simulink model "ED_PROJ"  (R2016a)
settings: Solver=VariableStepAuto  StartTime=0.0  StopTime=2  RelTol=1e-3
libraries: powerlib x12, simulink x1
settings Model: Creator=Deepak  LastModifiedBy=Deepak

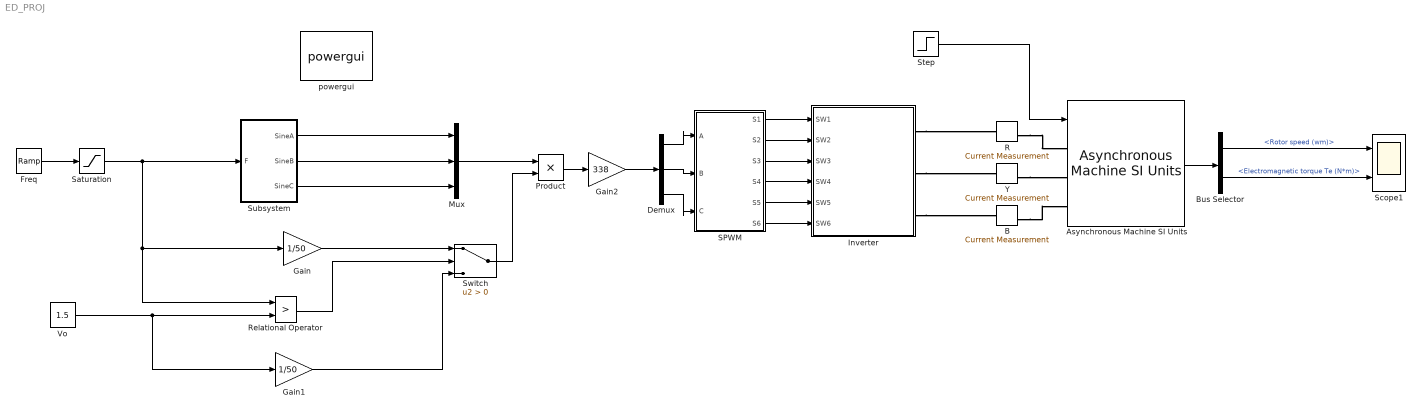
== system ED_PROJ ==
  Asynchronous Machine SI Units : powerlib/Machines/Asynchronous Machine SI Units  RotorType=Squirrel-cage  PresetModel=No  MechanicalLoad=Torque Tm  ShowDetailedParameters=on  ReferenceFrame=Rotor  Units=SI  MeasurementBus=off  NominalParameters=[1.845e+04 415 50]  Stator=[0.5968 0.0003495]  Rotor=[0.6258 0.005473]  Cage1=[0.4155 0.002066]  Cage2=[0.4168 0.0003495]  Lm=0.0354  Mechanical=[0.05 0.005879 2]  PolePairs=2  InitialConditions=[1 0 0 0 0 0 0 0]  SimulateSaturation=off  Saturation=[14.03593122, 27.81365428, 53.79336849, 72.68890987, 97.98006896, 148.6815601, 215.7428561, 302.9841135, 428.7778367 ; 230, 322, 414, 460, 506, 552, 598, 644, 690]  LoadFlowParameters=1492000  TsPowergui=0  TsBlock=-1  IterativeModel=Trapezoidal non iterative  IterativeDiscreteModel=Trapezoidal non iterative  Pmec=1.492e+006
  B : powerlib/Measurements/Current Measurement  PhasorSimulation=off  OutputType=Complex  PSBequivalent=0
  Bus Selector : BusSelector  OutputSignals=Mechanical.Rotor speed (wm),Mechanical.Electromagnetic torque Te (N*m)
  Demux : Demux  Outputs=3
  Freq : simulink/Sources/Ramp  slope=50  start=0  X0=0
  Gain : Gain  Gain=1/50
  Gain1 : Gain  Gain=1/50
  Gain2 : Gain  Gain=338
  Inverter : Subsystem
  Mux : Mux  Inputs=3
  Product : Product
  R : powerlib/Measurements/Current Measurement  PhasorSimulation=off  OutputType=Complex  PSBequivalent=0
  Relational Operator : RelationalOperator  Operator=>  OutDataTypeStr=boolean
  SPWM : Subsystem
  Saturation : Saturate  UpperLimit=50  LowerLimit=0
  Scope1 : Scope  NumInputPorts=2
  Step : Step  Time=10  Before=0.00001  After=5
  Subsystem : Subsystem
  Switch : Switch  Criteria=u2 > Threshold
  Vo : Constant  Value=1.5
  Y : powerlib/Measurements/Current Measurement  PhasorSimulation=off  OutputType=Complex  PSBequivalent=0
  powergui : powerlib/powergui  Priority=1  SimulationMode=Discrete  SolverType=Tustin/Backward Euler (TBE)  SampleTime=1e-06  frequency=60  SPID=off  DisableSnubberDevices=off  DisableRonSwitches=off  DisableVfSwitches=off  SwTol=0  DisplayEquations=off  Interpol=off  ExternalGateDelay=off  methode=off  Ts=10  FunctionMessages=off  echomessages=off  HookPort=off  EnableUseOfTLC=off  x0status=blocks  frequencyindice=0  Pbase=100e6  ErrMax=1e-4  Iterations=50  UnitsV=kV  UnitsW=MW  buscounter=0  RestoreLinks=warning  ResistiveCurrentMeasurement=off  Frange=[0:2:500]  Ylog=off  Xlog=on  ShowGrid=off  save=off  variable=ZData  structure=0  ZoomFFT=off  StartTime=0.0  cycles=1  DisplayStyle=1  fundamental=60  FreqAxis=off  MaxFrequency=1000  frequencyindicesteady=1  RmsSteady=1  display=off
  wires:
  Freq/1 -> Saturation/1
  Vo/1 -> Gain1/1, Relational Operator/2
  Saturation/1 -> Relational Operator/1, Gain/1, Subsystem/1(F)
  Relational Operator/1 -> Switch/2
  Gain/1 -> Switch/1
  Gain1/1 -> Switch/3
  Subsystem/1(SineA) -> Mux/1
  Subsystem/2(SineB) -> Mux/2
  Subsystem/3(SineC) -> Mux/3
  Mux/1 -> Product/1
  Switch/1 -> Product/2
  Product/1 -> Gain2/1
  Gain2/1 -> Demux/1
  Demux/2 -> SPWM/2(B)
  Demux/1 -> SPWM/1(A)
  Demux/3 -> SPWM/3(C)
  Asynchronous Machine SI Units/1 -> Bus Selector/1
  Step/1 -> Asynchronous Machine SI Units/1
  Bus Selector/1 -> Scope1/1  "<Rotor speed (wm)>"
  Bus Selector/2 -> Scope1/2  "<Electromagnetic torque Te (N*m)>"
  SPWM/1(S1) -> Inverter/1(SW1)
  SPWM/2(S2) -> Inverter/2(SW2)
  SPWM/3(S3) -> Inverter/3(SW3)
  SPWM/4(S4) -> Inverter/4(SW4)
  SPWM/5(S5) -> Inverter/5(SW5)
  SPWM/6(S6) -> Inverter/6(SW6)
  connections:
  R/RConn1 -- Asynchronous Machine SI Units/LConn1
  Y/RConn1 -- Asynchronous Machine SI Units/LConn2
  B/RConn1 -- Asynchronous Machine SI Units/LConn3
  Inverter/RConn1 -- R/LConn1
  Inverter/RConn2 -- Y/LConn1
  Inverter/RConn3 -- B/LConn1

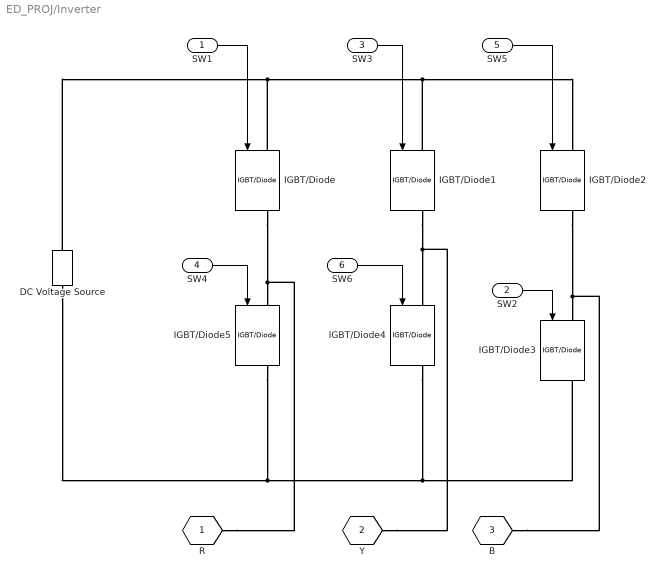
== system ED_PROJ/Inverter ==
  SW1 : Inport
  SW2 : Inport  Port=2
  SW3 : Inport  Port=3
  SW4 : Inport  Port=4
  SW5 : Inport  Port=5
  SW6 : Inport  Port=6
  DC Voltage Source : powerlib/Electrical Sources/DC Voltage Source  Amplitude=700  Measurements=None
  IGBT/Diode{,1..5} (6 alike) : powerlib/Power Electronics/IGBT//Diode  Ron=1e-3  Rs=1e5  Cs=inf  Measurements=on
  R : PMIOPort  Tag=PMCPort  Port=1  Side=Right
  Y : PMIOPort  Tag=PMCPort  Port=2  Side=Right
  B : PMIOPort  Tag=PMCPort  Port=3  Side=Right
  wires:
  SW1/1 -> IGBT/Diode/1
  SW5/1 -> IGBT/Diode2/1
  SW2/1 -> IGBT/Diode3/1
  SW3/1 -> IGBT/Diode1/1
  SW4/1 -> IGBT/Diode5/1
  SW6/1 -> IGBT/Diode4/1
  connections:
  DC Voltage Source/LConn1 -- IGBT/Diode5/RConn1 -- IGBT/Diode4/RConn1 -- IGBT/Diode3/RConn1
  IGBT/Diode/RConn1 -- R/RConn1 -- IGBT/Diode5/LConn1
  IGBT/Diode2/RConn1 -- B/RConn1 -- IGBT/Diode3/LConn1
  IGBT/Diode1/RConn1 -- Y/RConn1 -- IGBT/Diode4/LConn1
  DC Voltage Source/RConn1 -- IGBT/Diode2/LConn1 -- IGBT/Diode1/LConn1 -- IGBT/Diode/LConn1

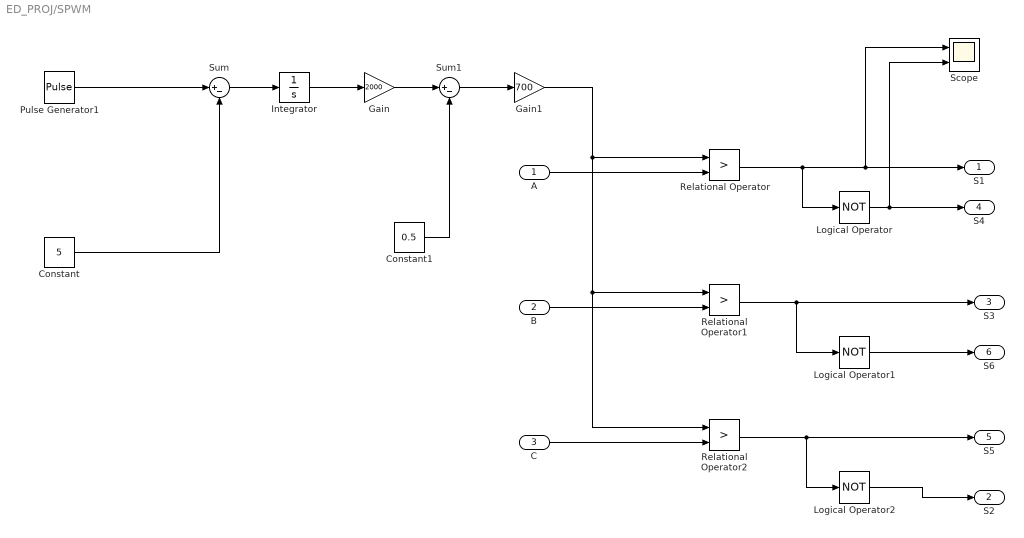
== system ED_PROJ/SPWM ==
  A : Inport
  B : Inport  Port=2
  C : Inport  Port=3
  Constant : Constant  Value=5
  Constant1 : Constant  Value=0.5
  Gain : Gain  Gain=2000
  Gain1 : Gain  Gain=700
  Integrator : Integrator
  Logical Operator : Logic  Operator=NOT  AllPortsSameDT=off  OutDataTypeStr=boolean
  Logical Operator1 : Logic  Operator=NOT  AllPortsSameDT=off  OutDataTypeStr=boolean
  Logical Operator2 : Logic  Operator=NOT  AllPortsSameDT=off  OutDataTypeStr=boolean
  Pulse Generator1 : DiscretePulseGenerator  PulseType=Time based  Amplitude=10  Period=2e-4  PulseWidth=50
  Relational Operator : RelationalOperator  Operator=>  OutDataTypeStr=boolean
  Relational Operator1 : RelationalOperator  Operator=>  OutDataTypeStr=boolean
  Relational Operator2 : RelationalOperator  Operator=>  OutDataTypeStr=boolean
  Scope : Scope  NumInputPorts=2
  Sum : Sum  Inputs=|+-
  Sum1 : Sum  Inputs=|+-
  S1 : Outport
  S2 : Outport  Port=2
  S3 : Outport  Port=3
  S4 : Outport  Port=4
  S5 : Outport  Port=5
  S6 : Outport  Port=6
  wires:
  Integrator/1 -> Gain/1
  Sum/1 -> Integrator/1
  Relational Operator1/1 -> S3/1, Logical Operator1/1
  B/1 -> Relational Operator1/2
  Logical Operator/1 -> S4/1, Scope/2
  Sum1/1 -> Gain1/1
  Pulse Generator1/1 -> Sum/1
  Constant/1 -> Sum/2
  Gain/1 -> Sum1/1
  Constant1/1 -> Sum1/2
  Relational Operator/1 -> S1/1, Scope/1, Logical Operator/1
  A/1 -> Relational Operator/2
  Gain1/1 -> Relational Operator2/1, Relational Operator1/1, Relational Operator/1
  C/1 -> Relational Operator2/2
  Relational Operator2/1 -> S5/1, Logical Operator2/1
  Logical Operator1/1 -> S6/1
  Logical Operator2/1 -> S2/1

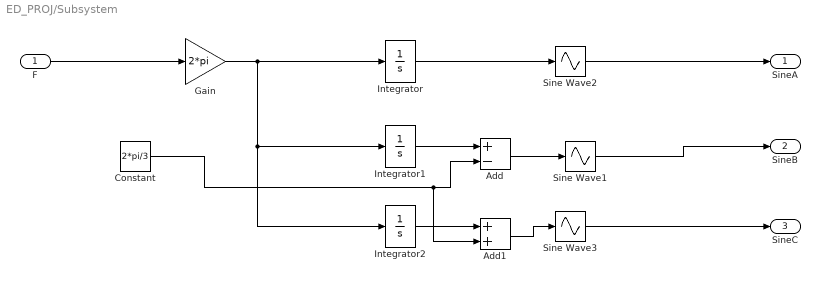
== system ED_PROJ/Subsystem ==
  F : Inport
  Add : Sum  Inputs=+-
  Add1 : Sum
  Constant : Constant  Value=2*pi/3
  Gain : Gain  Gain=2*pi
  Integrator : Integrator
  Integrator1 : Integrator
  Integrator2 : Integrator
  Sine Wave1 : Sin  TimeSource=Use external signal  SampleTime=0
  Sine Wave2 : Sin  TimeSource=Use external signal  SampleTime=0
  Sine Wave3 : Sin  TimeSource=Use external signal  SampleTime=0
  SineA : Outport
  SineB : Outport  Port=2
  SineC : Outport  Port=3
  wires:
  Integrator/1 -> Sine Wave2/1
  Add1/1 -> Sine Wave3/1
  F/1 -> Gain/1
  Integrator2/1 -> Add1/1
  Constant/1 -> Add1/2, Add/2
  Gain/1 -> Integrator1/1, Integrator2/1, Integrator/1
  Sine Wave3/1 -> SineC/1
  Sine Wave2/1 -> SineA/1
  Sine Wave1/1 -> SineB/1
  Integrator1/1 -> Add/1
  Add/1 -> Sine Wave1/1
